simulink model "ifir_dezim_1"  (Simulink 7.8)
settings: Solver=FixedStepDiscrete  SolverMode=SingleTasking  StartTime=0.0  StopTime=10.0  RelTol=1e-3
values from neighbouring files (symbols this model uses):
  h = firpm(64,f,m)    [CFIR_1.m]    (also in adapt_filter1.m = adaptfilt.lms(ni,mu); adapt_filter2.m = adaptfilt.blms(ni,mu,1,36); adaptiv_2.m = [1 2 3 4 5 6 7 8 9 10]; adaptiv_3.m = [1 2 3 4 5 6 7 8 9 10])
  L = 24    [G722_1.m]    (also in adaptiv_2.m = length(h); adaptiv_3.m = length(h); audio_test1.m = 64; audio_test2.m = 64)
  Ts = 1/fs    (= 6.25e-05)    [G722_1.m]    (also in adaptiv_2.m = 0.001; adaptiv_3.m = 0.001; adaptiv_4.m = 0.001; adaptiv_5.m = 0.001)
undefined symbols (not defined in the file or in its folder): himage, hsig
libraries: dspsigops x2
settings Model: Creator=svenhoffmann  LastModifiedBy=josef  ExtModeAutoUpdateStatusClock=off
settings OptimizationCC: InlineInvariantSignals=on  InitFltsAndDblsToZero=on
settings DebuggingCC: SaveWithParameterizedLinksMsg=none  SignalResolutionControl=TryResolveAllWithWarning  MultiTaskDSMMsg=warning  MultiTaskCondExecSysMsg=none  FcnCallInpInsideContextMsg=Use local settings  StrictBusMsg=None
settings RTWCC: IncludeERTFirstTime=on
settings GRTTargetCC: TargetFcnLib=ansi_tfl_tmw.mat

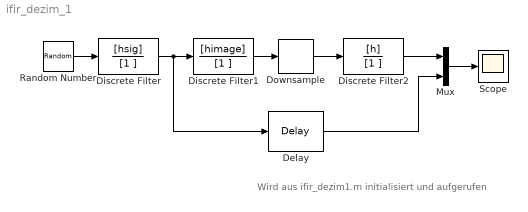
== system ifir_dezim_1 ==
  note: Wird aus ifir_dezim1.m initialisiert und aufgerufen
  Delay : dspsigops/Delay  InputProcessing=Inherited (this choice will be removed - see release notes)  dly_unit=Samples  delay=delay  ic_detail=off  dif_ic_for_ch=off  dif_ic_for_dly=off  ic=0  reset_popup=None
  Discrete Filter : DiscreteFilter  Numerator=[hsig]  Denominator=[1 ]  SampleTime=Ts
  Discrete Filter1 : DiscreteFilter  Numerator=[himage]  Denominator=[1 ]  SampleTime=Ts
  Discrete Filter2 : DiscreteFilter  Numerator=[h]  Denominator=[1 ]  SampleTime=Ts*L
  Downsample : dspsigops/Downsample  N=L  phase=0  InputProcessing=Inherited (this choice will be removed - see release notes)  RateOptions=Enforce single-rate processing  smode=Allow multirate  fmode=Maintain input frame size  ic=0
  Mux : Mux  Inputs=2
  Random Number : RandomNumber  SampleTime=Ts
  Scope : Scope
      settings: TimeRange=1
  wires:
  Random Number/1 -> Discrete Filter/1
  Discrete Filter/1 -> Discrete Filter1/1, Delay/1
  Discrete Filter1/1 -> Downsample/1
  Downsample/1 -> Discrete Filter2/1
  Discrete Filter2/1 -> Mux/1
  Delay/1 -> Mux/2
  Mux/1 -> Scope/1
